simulink model "Part1_2019a"  (R2019a)
settings: Solver=ode45  StartTime=0.0  StopTime=50  FixedStep=Ts  RelTol=1e-3  EnableMultiTasking=on
values from neighbouring files (symbols this model uses):
  alfa1 = .2    (= 0.2)    [parameters.m]
  alfa2 = .2    (= 0.2)    [parameters.m]
  b1 = 0.1    [parameters.m]
  b2 = 0.1    [parameters.m]
  b3_nom = 0.1    [parameters.m]
  b4_nom = 0.1    [parameters.m]
  b5 = 0.1    [parameters.m]
  C_D_Re_GNARC = C_C_Re    [start_up.m]
  D_D_Re_GNARC = D_C_Re    [start_up.m]
  k1 = 0.15    [parameters.m]
  k3_nom = .1    (= 0.1)    [parameters.m]
  k4_nom = .1    (= 0.1)    [parameters.m]
  m1 = 1    [parameters.m]
  m2 = 1    [parameters.m]
  m3 = 1    [parameters.m]
  m4 = 1    [parameters.m]
  Ts = 0.001    [parameters.m]
undefined symbols (not defined in the file or in its folder): A_D_Re_GNARC, B_D_Re_GNARC
libraries: simulink x4
settings Model: Creator=VAHiD  LastModifiedBy=zhy
settings DataIOCC: LimitDataPoints=on  SaveFormat=Array  ReturnWorkspaceOutputs=off
settings OptimizationCC: ExpressionDepthLimit=2147483647  LifeSpan=inf
settings DebuggingCC: UnderspecifiedInitializationDetection=Classic  MergeDetectMultiDrivingBlocksExec=none  SolverPrmCheckMsg=warning  FcnCallInpInsideContextMsg=warning  StateNameClashWarn=warning  SFUnexpectedBacktrackingDiag=warning  SFNoUnconditionalDefaultTransitionDiag=warning  SFExecutionAtInitializationDiag=none  ArithmeticOperatorsInVariantConditions=warning
settings HardwareCC: ProdBitPerPointer=32  ProdBitPerSizeT=32  ProdBitPerPtrDiffT=32  ProdLargestAtomicFloat=None  ProdIntDivRoundTo=Undefined  ProdEndianess=Unspecified  ProdWordSize=32  ProdHWDeviceType=32-bit Generic
settings ModelReferenceCC: PropagateSignalLabelsOutOfModel=off
settings SFSimCC: SimUseLocalCustomCode=off
settings RTWCC: RTWUseLocalCustomCode=off
settings CodeAppCC: StateflowObjectComments=on
settings GRTTargetCC: TargetLangStandard=C89/C90 (ANSI)  GeneratePreprocessorConditionals=Disable all  CombineOutputUpdateFcns=off  GRTInterface=on
settings ConfigComp: CovMetricSettings=dw  CovHtmlReporting=on  CovSaveCumulativeToWorkspaceVar=on  CovSaveSingleToWorkspaceVar=on  CovExternalEMLEnable=off

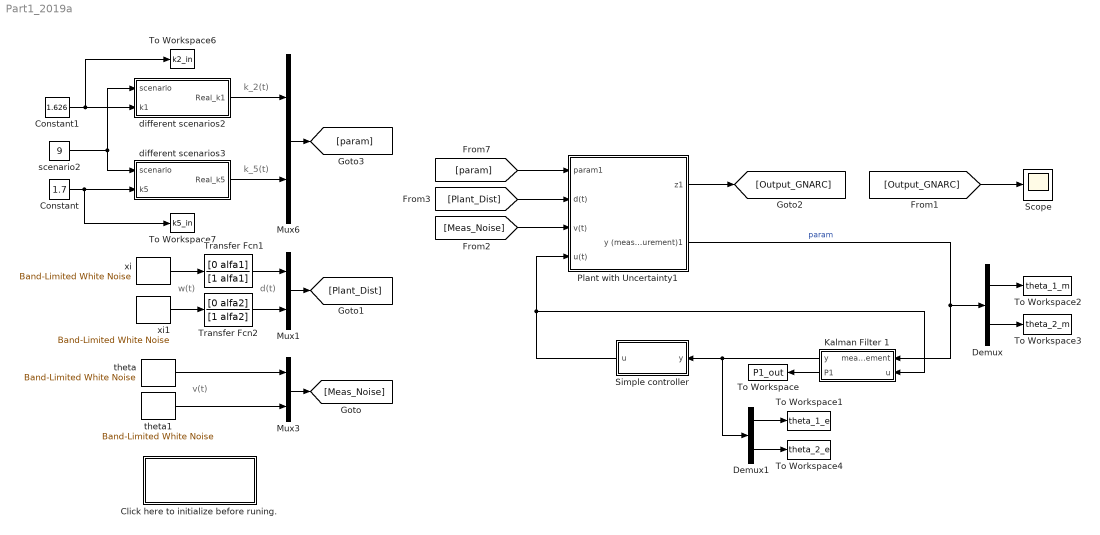
== system Part1_2019a ==
  note: w(t)
  note: v(t)
  note: d(t)
  note: k_2(t)
  note: k_5(t)
  Click here to initialize before runing. : Subsystem
      settings: OpenFcn=start_up
      mask Display: disp('Load\Parameters')
  Constant : Constant  Value=1.7
  Constant1 : Constant  Value=1.626
  Demux : Demux  Outputs=2
  Demux1 : Demux  Outputs=2
  Kalman Filter 1 : Subsystem
  Mux1 : Mux  Inputs=2
  Mux3 : Mux  Inputs=2
  Mux6 : Mux  Inputs=2
  Plant with Uncertainty1 : Subsystem
  Scope : Scope
  Simple controller : Subsystem
  To Workspace : ToWorkspace  VariableName=P1_out  SampleTime=-1
      settings: Save2DSignal=2-D array (concatenate along first dimension)
  To Workspace1 : ToWorkspace  VariableName=theta_1_e  SaveFormat=Timeseries  SampleTime=-1
  To Workspace2 : ToWorkspace  VariableName=theta_1_m  SaveFormat=Timeseries  SampleTime=-1
  To Workspace3 : ToWorkspace  VariableName=theta_2_m  SaveFormat=Timeseries  SampleTime=-1
  To Workspace4 : ToWorkspace  VariableName=theta_2_e  SaveFormat=Timeseries  SampleTime=-1
  To Workspace6 : ToWorkspace  VariableName=k2_in  SaveFormat=Timeseries  SampleTime=-1
  To Workspace7 : ToWorkspace  VariableName=k5_in  SaveFormat=Timeseries  SampleTime=-1
  Transfer Fcn1 : TransferFcn  Numerator=[0 alfa1]  Denominator=[1 alfa1]
  Transfer Fcn2 : TransferFcn  Numerator=[0 alfa2]  Denominator=[1 alfa2]
  different scenarios2 : Subsystem
  different scenarios3 : Subsystem
  scenario2 : Constant  Value=9
  theta : simulink/Sources/Band-Limited White Noise  Cov=TH1  Ts=Ts  seed=1
  theta1 : simulink/Sources/Band-Limited White Noise  Cov=TH2  Ts=Ts  seed=2
  xi : simulink/Sources/Band-Limited White Noise  Cov=XI1  Ts=Ts  seed=3
  xi1 : simulink/Sources/Band-Limited White Noise  Cov=XI2  Ts=Ts  seed=4
  wires:
  Mux3/1 -> [Meas_Noise]
  theta/1 -> Mux3/1
  theta1/1 -> Mux3/2
  Mux1/1 -> [Plant_Dist]
  xi/1 -> Transfer Fcn1/1
  xi1/1 -> Transfer Fcn2/1
  Transfer Fcn1/1 -> Mux1/1
  Transfer Fcn2/1 -> Mux1/2
  scenario2/1 -> different scenarios2/1(scenario), different scenarios3/1(scenario)
  different scenarios3/1(Real_k5) -> Mux6/2
  different scenarios2/1(Real_k1) -> Mux6/1
  Mux6/1 -> [param]
  [param] -> Plant with Uncertainty1/1(param1)
  [Plant_Dist] -> Plant with Uncertainty1/2(d(t))
  [Meas_Noise] -> Plant with Uncertainty1/3(v(t))
  Plant with Uncertainty1/1(z1) -> [Output_GNARC]
  [Output_GNARC] -> Scope/1
  Plant with Uncertainty1/2(y (measurement)1) -> Demux/1, Kalman Filter 1/1(measurement)  "param"
  Kalman Filter 1/2(P1) -> To Workspace/1
  Constant1/1 -> To Workspace6/1, different scenarios2/2(k1)
  Constant/1 -> To Workspace7/1, different scenarios3/2(k5)
  Simple controller/1(u) -> Plant with Uncertainty1/4(u(t)), Kalman Filter 1/2(u)
  Kalman Filter 1/1(y) -> Demux1/1, Simple controller/1(y)
  Demux/1 -> To Workspace2/1
  Demux/2 -> To Workspace3/1
  Demux1/1 -> To Workspace1/1
  Demux1/2 -> To Workspace4/1

== system Part1_2019a/Click here to initialize before runing. ==

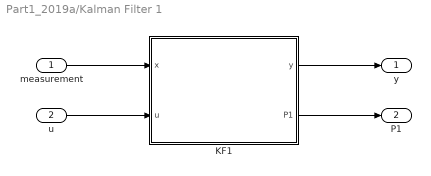
== system Part1_2019a/Kalman Filter 1 ==
  measurement : Inport
  u : Inport  Port=2
  KF1 : MATLAB Function  TreatAsAtomicUnit=on
  y : Outport
  P1 : Outport  Port=2
  wires:
  u/1 -> KF1/2(u)
  measurement/1 -> KF1/1(x)
  KF1/1(y) -> y/1
  KF1/2(P1) -> P1/1

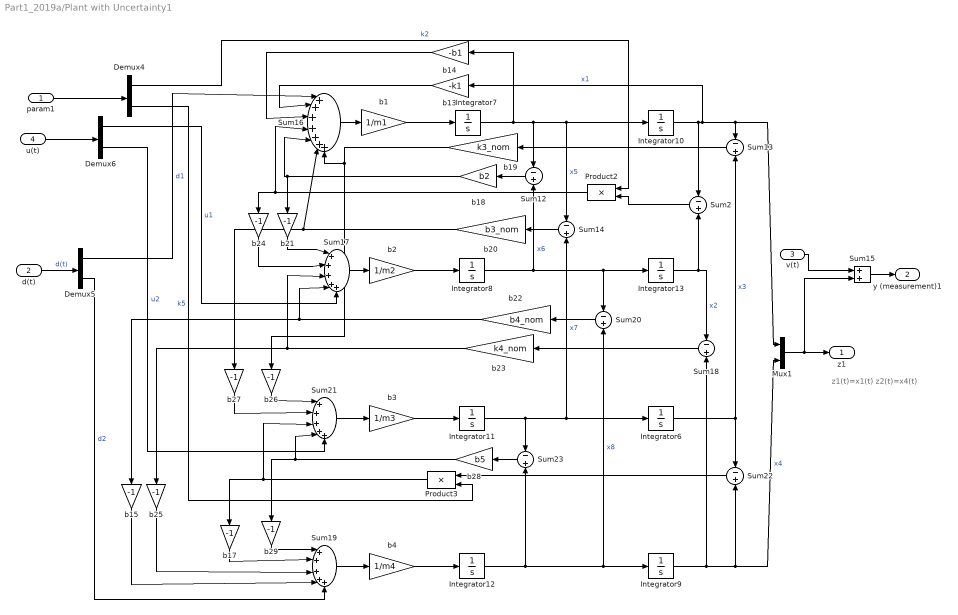
== system Part1_2019a/Plant with Uncertainty1 ==
  note: z1(t)=x1(t)
      | z2(t)=x4(t)
  param1 : Inport
  d(t) : Inport  Port=2
  v(t) : Inport  Port=3
  u(t) : Inport  Port=4
  Demux4 : Demux  Outputs=2
  Demux5 : Demux  Outputs=2
  Demux6 : Demux  Outputs=2
  Integrator{6..13} (8 alike) : Integrator
  Mux1 : Mux  Inputs=2
  Product2 : Product  SaturateOnIntegerOverflow=on  InputSameDT=on  OutDataTypeStr=Inherit: Same as first input
  Product3 : Product  SaturateOnIntegerOverflow=on  InputSameDT=on  OutDataTypeStr=Inherit: Same as first input
  Sum{2,12..14,18,20,22..23} (8 alike) : Sum  Inputs=-+  SaturateOnIntegerOverflow=on  InputSameDT=on  OutDataTypeStr=Inherit: Same as first input
  Sum15 : Sum  SaturateOnIntegerOverflow=on  InputSameDT=on  OutDataTypeStr=Inherit: Same as first input
  Sum16 : Sum  Inputs=|+++++++  SaturateOnIntegerOverflow=on  InputSameDT=on  OutDataTypeStr=Inherit: Same as first input
  Sum17 : Sum  Inputs=|+++++  SaturateOnIntegerOverflow=on  InputSameDT=on  OutDataTypeStr=Inherit: Same as first input
  Sum19 : Sum  Inputs=|+++++  SaturateOnIntegerOverflow=on  InputSameDT=on  OutDataTypeStr=Inherit: Same as first input
  Sum21 : Sum  Inputs=|+++++  SaturateOnIntegerOverflow=on  InputSameDT=on  OutDataTypeStr=Inherit: Same as first input
  b1 : Gain  Gain=1/m1  SaturateOnIntegerOverflow=on  OutDataTypeStr=Inherit: Same as input  ParamDataTypeStr=Inherit: Same as input
  b13 : Gain  Gain=-k1  SaturateOnIntegerOverflow=on  OutDataTypeStr=Inherit: Same as input  ParamDataTypeStr=Inherit: Same as input
  b14 : Gain  Gain=-b1  SaturateOnIntegerOverflow=on  OutDataTypeStr=Inherit: Same as input  ParamDataTypeStr=Inherit: Same as input
  b{15,17,21,24..27,29} (8 alike) : Gain  Gain=-1  SaturateOnIntegerOverflow=on  OutDataTypeStr=Inherit: Same as input  ParamDataTypeStr=Inherit: Same as input
  b18 : Gain  Gain=b2  SaturateOnIntegerOverflow=on  OutDataTypeStr=Inherit: Same as input  ParamDataTypeStr=Inherit: Same as input
  b19 : Gain  Gain=k3_nom  SaturateOnIntegerOverflow=on  OutDataTypeStr=Inherit: Same as input  ParamDataTypeStr=Inherit: Same as input
  b2 : Gain  Gain=1/m2  SaturateOnIntegerOverflow=on  OutDataTypeStr=Inherit: Same as input  ParamDataTypeStr=Inherit: Same as input
  b20 : Gain  Gain=b3_nom  SaturateOnIntegerOverflow=on  OutDataTypeStr=Inherit: Same as input  ParamDataTypeStr=Inherit: Same as input
  b22 : Gain  Gain=b4_nom  SaturateOnIntegerOverflow=on  OutDataTypeStr=Inherit: Same as input  ParamDataTypeStr=Inherit: Same as input
  b23 : Gain  Gain=k4_nom  SaturateOnIntegerOverflow=on  OutDataTypeStr=Inherit: Same as input  ParamDataTypeStr=Inherit: Same as input
  b28 : Gain  Gain=b5  SaturateOnIntegerOverflow=on  OutDataTypeStr=Inherit: Same as input  ParamDataTypeStr=Inherit: Same as input
  b3 : Gain  Gain=1/m3  SaturateOnIntegerOverflow=on  OutDataTypeStr=Inherit: Same as input  ParamDataTypeStr=Inherit: Same as input
  b4 : Gain  Gain=1/m4  SaturateOnIntegerOverflow=on  OutDataTypeStr=Inherit: Same as input  ParamDataTypeStr=Inherit: Same as input
  z1 : Outport
  y (measurement)1 : Outport  Port=2
  wires:
  Sum15/1 -> y (measurement)1/1
  v(t)/1 -> Sum15/1
  param1/1 -> Demux4/1
  Mux1/1 -> Sum15/2, z1/1
  d(t)/1 -> Demux5/1  "d(t)"
  u(t)/1 -> Demux6/1
  b25/1 -> Sum19/3
  b15/1 -> Sum19/4
  Demux5/2 -> Sum19/5  "d2"
  Integrator7/1 -> b14/1, Sum12/1, Integrator10/1, Sum14/1  "x5"
  Integrator10/1 -> b13/1, Sum13/1, Mux1/1, Sum2/1  "x1"
  Integrator8/1 -> Sum12/2, Integrator13/1, Sum20/1  "x6"
  Integrator11/1 -> Integrator6/1, Sum14/2, Sum23/1  "x7"
  Integrator12/1 -> Integrator9/1, Sum20/2, Sum23/2  "x8"
  Demux5/1 -> Sum16/1  "d1"
  b13/1 -> Sum16/2
  b14/1 -> Sum16/3
  Integrator13/1 -> Sum2/2, Sum18/1  "x2"
  Sum2/1 -> Product2/2
  Demux4/1 -> Product2/1  "k2"
  Sum12/1 -> b18/1
  b18/1 -> Sum16/5, b21/1
  Integrator6/1 -> Sum13/2, Sum22/1  "x3"
  Sum13/1 -> b19/1
  Sum14/1 -> b20/1
  b20/1 -> Sum16/6, b27/1
  Sum16/1 -> b1/1
  Product2/1 -> Sum16/4, b24/1
  Integrator9/1 -> Sum18/2, Sum22/2, Mux1/2  "x4"
  Sum18/1 -> b23/1
  b23/1 -> Sum17/3, b25/1
  Sum17/1 -> b2/1
  Sum20/1 -> b22/1
  b22/1 -> Sum17/4, b15/1
  b21/1 -> Sum17/1
  b24/1 -> Sum17/2
  Demux6/1 -> Sum17/5  "u1"
  Sum21/1 -> b3/1
  b19/1 -> Sum16/7, b26/1
  b26/1 -> Sum21/1
  b27/1 -> Sum21/2
  Sum22/1 -> Product3/1
  Product3/1 -> Sum21/3, b17/1
  Demux4/2 -> Product3/2  "k5"
  Sum23/1 -> b28/1
  b28/1 -> Sum21/4, b29/1
  Demux6/2 -> Sum21/5  "u2"
  Sum19/1 -> b4/1
  b17/1 -> Sum19/2
  b29/1 -> Sum19/1
  b1/1 -> Integrator7/1
  b2/1 -> Integrator8/1
  b3/1 -> Integrator11/1
  b4/1 -> Integrator12/1

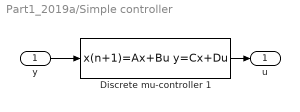
== system Part1_2019a/Simple controller ==
  y : Inport
  Discrete mu-controller 1 : DiscreteStateSpace  Description=disp('sss')  A=A_D_Re_GNARC  B=B_D_Re_GNARC  C=C_D_Re_GNARC  D=D_D_Re_GNARC  SampleTime=Ts
  u : Outport
  wires:
  y/1 -> Discrete mu-controller 1/1
  Discrete mu-controller 1/1 -> u/1

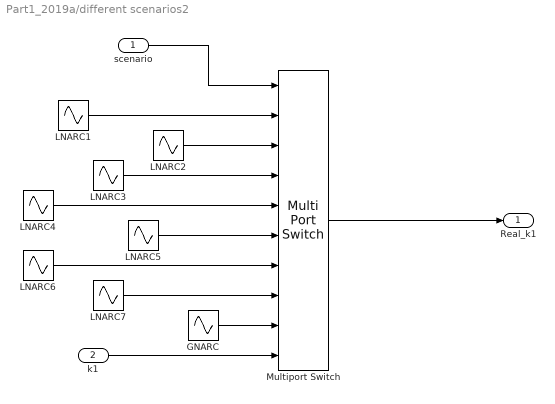
== system Part1_2019a/different scenarios2 ==
  scenario : Inport
  k1 : Inport  Port=2
  GNARC : Sin  Amplitude=.75  Bias=1  Frequency=2*pi/700  Phase=-pi/2  SampleTime=0
  LNARC1 : Sin  Amplitude=.875  Bias=1.625  Frequency=2*pi/700  Phase=-pi/2  SampleTime=0
  LNARC2 : Sin  Amplitude=.55/2  Bias=.775  Frequency=2*pi/700  Phase=-pi/2  SampleTime=0
  LNARC3 : Sin  Amplitude=.75/2  Bias=1.4250  Frequency=2*pi/700  Phase=-pi/2  SampleTime=0
  LNARC4 : Sin  Amplitude=.15/2  Bias=.325  Frequency=2*pi/700  Phase=-pi/2  SampleTime=0
  LNARC5 : Sin  Amplitude=.15  Bias=.55  Frequency=2*pi/700  Phase=-pi/2  SampleTime=0
  LNARC6 : Sin  Amplitude=.45/2  Bias=.925  Frequency=2*pi/700  Phase=-pi/2  SampleTime=0
  LNARC7 : Sin  Amplitude=.30  Bias=1.45  Frequency=2*pi/700  Phase=-pi/2  SampleTime=0
  Multiport Switch : MultiPortSwitch  Inputs=9
  Real_k1 : Outport
  wires:
  Multiport Switch/1 -> Real_k1/1
  scenario/1 -> Multiport Switch/1
  LNARC3/1 -> Multiport Switch/4
  LNARC6/1 -> Multiport Switch/7
  LNARC7/1 -> Multiport Switch/8
  LNARC5/1 -> Multiport Switch/6
  LNARC4/1 -> Multiport Switch/5
  LNARC1/1 -> Multiport Switch/2
  LNARC2/1 -> Multiport Switch/3
  k1/1 -> Multiport Switch/10
  GNARC/1 -> Multiport Switch/9

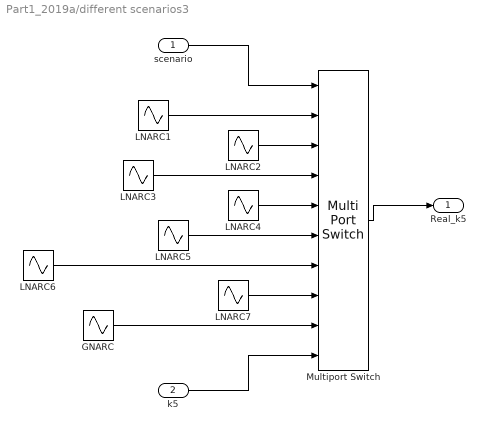
== system Part1_2019a/different scenarios3 ==
  scenario : Inport
  k5 : Inport  Port=2
  GNARC : Sin  Amplitude=1.6  Bias=1.8  Frequency=2*pi/700  Phase=-pi/2  SampleTime=0
  LNARC1 : Sin  Amplitude=.8  Bias=1.7  Frequency=2*pi/700  Phase=-3*pi/2  SampleTime=0
  LNARC2 : Sin  Amplitude=.8  Bias=2.6  Frequency=2*pi/700  Phase=-pi/2  SampleTime=0
  LNARC3 : Sin  Amplitude=.8  Bias=2.6  Frequency=2*pi/700  Phase=-pi/2  SampleTime=0
  LNARC{4..7} (4 alike) : Sin  Amplitude=.8  Bias=1  Frequency=2*pi/700  Phase=-pi/2  SampleTime=0
  Multiport Switch : MultiPortSwitch  Inputs=9
  Real_k5 : Outport
  wires:
  LNARC5/1 -> Multiport Switch/6
  LNARC7/1 -> Multiport Switch/8
  LNARC6/1 -> Multiport Switch/7
  LNARC3/1 -> Multiport Switch/4
  scenario/1 -> Multiport Switch/1
  Multiport Switch/1 -> Real_k5/1
  k5/1 -> Multiport Switch/10
  GNARC/1 -> Multiport Switch/9
  LNARC1/1 -> Multiport Switch/2
  LNARC2/1 -> Multiport Switch/3
  LNARC4/1 -> Multiport Switch/5

== matlab function Part1_2019a/Kalman Filter 1/KF1 ==
  settings: updateMethod=DISCRETE  sampleTime=0.001
  data: x input; y output; u input; P1 output
function [y,P1] = KF_disc(x,u)

persistent P_bar;
persistent x_bar;
persistent P_hat;
persistent x_hat;

if isempty(P_bar)
    P_bar = zeros(10);
    x_bar = zeros(10,1);
    P_hat = zeros(10);
    x_hat = zeros(10,1);
end
    
k1=0.15; k2=1.626; k3=0.1; k4=0.1; k5=1.7;
b1=0.1;  b2=0.1; b3=0.1; b4=0.1; b5 =0.1;
J = 1;
A = [ 
    0 0 0 0 1 0 0 0 0 0;
    0 0 0 0 0 1 0 0 0 0;
    0 0 0 0 0 0 1 0 0 0;
    0 0 0 0 0 0 0 1 0 0;
    -(k1+k2+k3)/J k2/J k3/J 0 -(b1+b2+b3)/J b2/J b3/J 0 1/J 0;
    k2/J -(k2+k4)/J 0 k4/J b2/J -(b2+b4)/J 0 b4/J 0 0;
    k3/J 0 -(k3+k5)/J k5/J b3/J 0 -(b3+b5)/J b5/J 0 0;
    0 k4/J k5/J -(k4+k5)/J 0 b4/J b5/J -(b4+b5)/J 0 1/J;
    0 0 0 0 0 0 0 0 -0.2 0;
    0 0 0 0 0 0 0 0 0 -0.2
    ];
B = [0 0;0 0;0 0;0 0;0 0;1/J 0;0 1/J;0 0;0 0;0 0];
G = [0 0; 0 0; 0 0; 0 0; 0 0; 0 0; 0 0; 0 0; 0.2 0; 0 0.2];
C = [1 0 0 0 0 0 0 0 0 0;
     0 0 0 1 0 0 0 0 0 0];

 % Design covariance matrices 
R_c = diag([1e-6 1e-6]);
Q_c = diag([1 11]);

%% discrete matrix and parameters
Ts=0.001;
Phi = eye(10) + Ts*A;
Delta = inv(A)*(Phi-eye(10))*B;
Gamma = inv(A)*(Phi-eye(10))*G;
R_d = R_c/Ts;
Q_d = zeros(10,10);
Q_d(9,9) = 1e-3*0.04;
Q_d(10,10) = 1e-3*0.4399;

%% Kalman Filter
% Gain
K = P_bar*C'*inv(C*P_bar*C'+R_d);

x_hat = x_bar + K*(x - C*x_bar);
P_hat = (eye(10)- K*C)*P_bar*(eye(10)- K*C)'+ K*R_d*K';

x_bar = Phi*x_hat+Delta*u;
% P_bar = Phi*P_hat*Phi'+Gamma*Q_d*Gamma';
P_bar = Phi*P_hat*Phi'+ Q_d;
P1 = P_hat;
y = [x_hat(1); x_hat(4)];
